simulink model "IIR122"  (Simulink 7.9)
settings: Solver=FixedStepDiscrete  StartTime=0.0  StopTime=10.0  RelTol=1e-3
values from neighbouring files (symbols this model uses):
  G = 3/4    (= 0.75)    [IIRFrequencyResponse.m]    (also in createFIR.m = 0.25; createIIR.m; lab122freqresponseIIR.m)
libraries: simulink x1, dspsigops x1
settings Model: Creator=llugos  LastModifiedBy=llugos

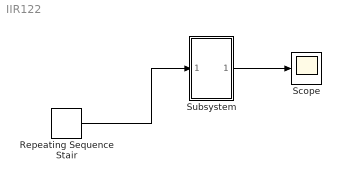
== system IIR122 ==
  Repeating Sequence Stair : simulink/Sources/Repeating Sequence Stair  OutValues=[3 1 4 2 1].'  tsamp=-1  OutMin=[]  OutMax=[]  OutDataTypeStr=double  OutputDataTypeScalingMode=double  OutDataType=fixdt(0,8)  ConRadixGroup=Best Precision: Vector-wise  OutScaling=2^-12
  Scope : Scope
  Subsystem : Subsystem
  wires:
  Repeating Sequence Stair/1 -> Subsystem/1(In1)
  Subsystem/1(Out1) -> Scope/1

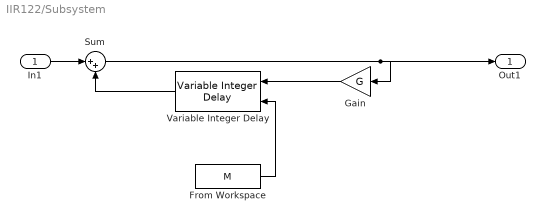
== system IIR122/Subsystem ==
  In1 : Inport
  From Workspace : FromWorkspace  VariableName=M  SampleTime=1  OutputAfterFinalValue=Holding final value
  Gain : Gain  Gain=G
  Sum : Sum  Inputs=|++
  Variable Integer Delay : dspsigops/Variable Integer Delay  dmax=100  InputProcessing=Columns as channels (frame based)  ic=0  noDFT=off
  Out1 : Outport
  wires:
  Gain/1 -> Variable Integer Delay/1
  From Workspace/1 -> Variable Integer Delay/2
  Variable Integer Delay/1 -> Sum/2
  Sum/1 -> Gain/1, Out1/1
  In1/1 -> Sum/1
